simulink model "ForwardDynamics_harmonic_sine"  (Simulink 7.9)
settings: Solver=ode45  StartTime=0.0  StopTime=1  RelTol=1e-3
settings Model: Creator=gwu  LastModifiedBy=gwu
settings RTWCC: TargetLang=C++

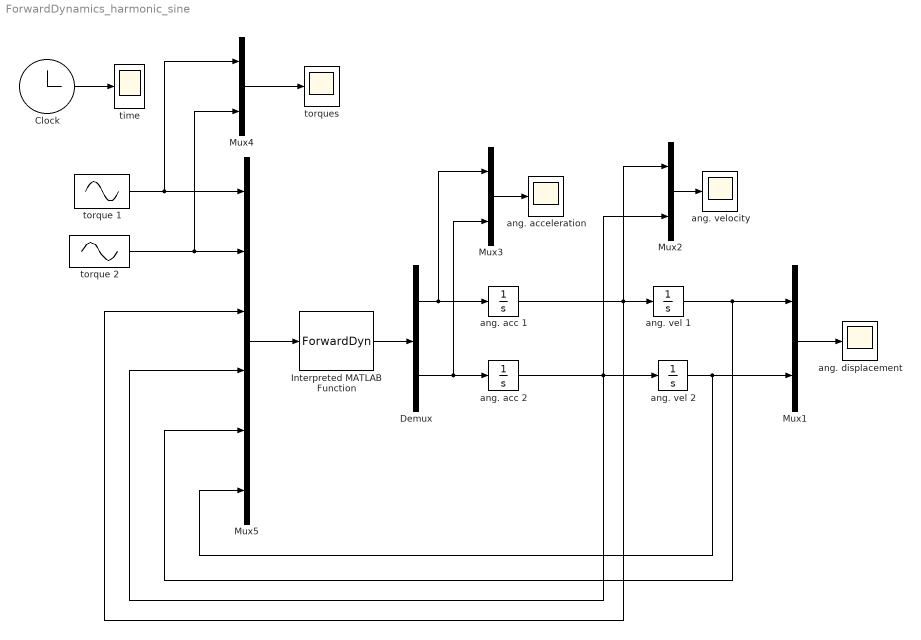
== system ForwardDynamics_harmonic_sine ==
  Clock : Clock
  Demux : Demux  Outputs=2
  Interpreted MATLAB Function : MATLABFcn  MATLABFcn=ForwardDyn
  Mux{1..4} (4 alike) : Mux  Inputs=2
  Mux5 : Mux  Inputs=6
  ang. acc 1 : Integrator
  ang. acc 2 : Integrator
  ang. acceleration : Scope
      settings: SaveName=ScopeData4
  ang. displacement : Scope
      settings: SaveName=ScopeData2
  ang. vel 1 : Integrator
  ang. vel 2 : Integrator
  ang. velocity : Scope
      settings: SaveName=ScopeData3
  time : Scope
      settings: SaveName=ScopeData5
  torque 1 : Sin  Amplitude=10  Frequency=pi  SampleTime=0
  torque 2 : Sin  Amplitude=5  Frequency=3*pi  SampleTime=0
  torques : Scope
      settings: SaveName=ScopeData6
  wires:
  ang. acc 1/1 -> ang. vel 1/1, Mux2/1, Mux5/3
  ang. vel 1/1 -> Mux1/1, Mux5/5
  ang. vel 2/1 -> Mux1/2, Mux5/6
  ang. acc 2/1 -> ang. vel 2/1, Mux2/2, Mux5/4
  torque 1/1 -> Mux4/1, Mux5/1
  torque 2/1 -> Mux4/2, Mux5/2
  Interpreted MATLAB Function/1 -> Demux/1
  Demux/1 -> ang. acc 1/1, Mux3/1
  Demux/2 -> ang. acc 2/1, Mux3/2
  Mux1/1 -> ang. displacement/1
  Mux2/1 -> ang. velocity/1
  Mux3/1 -> ang. acceleration/1
  Clock/1 -> time/1
  Mux4/1 -> torques/1
  Mux5/1 -> Interpreted MATLAB Function/1
